simulink model "EjercPid"  (R2015a)
settings: Solver=ode4  StartTime=0.0  StopTime=10  RelTol=1e-3
values from neighbouring files (symbols this model uses):
  b = [1 2 0]'    [Espacio_d_Estados.m]
  k = place(n1,b1,pc)    [dinam19.m]    (also in dinam20.m = place(A,B,pc))
  m = .5    (= 0.5)    [dinam20.m]    (also in dinam21.m; dinam22.m; vparachute.m)
settings Model: Creator=HP  LastModifiedBy=HP

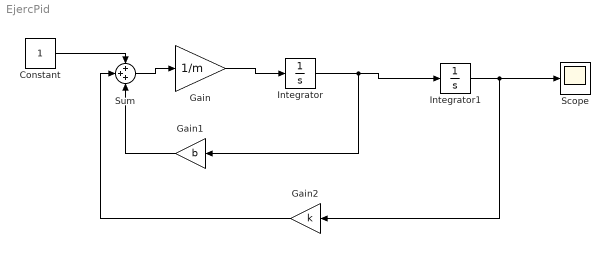
== system EjercPid ==
  Constant : Constant  VectorParams1D=off
  Gain : Gain  Gain=1/m
  Gain1 : Gain  Gain=b
  Gain2 : Gain  Gain=k
  Integrator : Integrator
  Integrator1 : Integrator
  Scope : Scope
  Sum : Sum  Inputs=+++
  wires:
  Sum/1 -> Gain/1
  Gain/1 -> Integrator/1
  Integrator1/1 -> Gain2/1, Scope/1
  Constant/1 -> Sum/1
  Integrator/1 -> Gain1/1, Integrator1/1
  Gain1/1 -> Sum/3
  Gain2/1 -> Sum/2
